simulink model "om2"  (Simulink 7.2)
(part 3 of 6)

      | Usage:                                                                                                                                                                                                                                    
      | Name the part with the desired filter module name.
      settings: AttributesFormatString=%<Tag>
  Y1_I : cdsFilt/Subsystem  Tag=cdsFilt  Description=|  SystemSampleTime=-1
      | Purpose:                                                                                                                                                                                                                                  
      | Standard CDS IIR filter module.                                                                                                                                                                                                           
      |                                                                                                                                                                                                                                           
      | Operation:                                                                                                                                                                                                                                
      | Consists of 10 second order section IIR filters, plus a ramped gain stage. In FE code, also provides pre-defined test points and excitation channel inputs. The filter coefficients are defined in the LIGO system using the 'foton' tool.
      |                                                                                                                                                                                                                                           
      | Usage:                                                                                                                                                                                                                                    
      | Name the part with the desired filter module name.
      settings: AttributesFormatString=%<Tag>
  Y1_MOUT : cdsEpicsOut/Subsystem  Tag=cdsEpicsOutput  Description=|  SystemSampleTime=-1
      | Purpose:                                          
      | Output a FE signal to an EPICS channel.           
      |                                                   
      | Operation:                                        
      | Takes input value and passes it to EPICS record.  
      |                                                   
      | Usage:                                            
      | Name the part with the desired EPICS rrecord name.
      settings: AttributesFormatString=%<Tag>
  Y1_OSC : cdsOsc/Subsystem  Tag=cdsOsc  Description=Oscillator  SystemSampleTime=-1
      settings: AttributesFormatString=%<Tag>
  Y1_OSC1 : cdsOsc/Subsystem  Tag=cdsOsc  Description=Oscillator  SystemSampleTime=-1
      settings: AttributesFormatString=%<Tag>
  Y1_PHASE : cdsPhaseDeg/Subsystem  Tag=cdsPhaseDeg  Description=Phase Rotator  SystemSampleTime=-1
      settings: AttributesFormatString=%<Tag>
  Y1_Q : cdsFilt/Subsystem  Tag=cdsFilt  Description=|  SystemSampleTime=-1
      | Purpose:                                                                                                                                                                                                                                  
      | Standard CDS IIR filter module.                                                                                                                                                                                                           
      |                                                                                                                                                                                                                                           
      | Operation:                                                                                                                                                                                                                                
      | Consists of 10 second order section IIR filters, plus a ramped gain stage. In FE code, also provides pre-defined test points and excitation channel inputs. The filter coefficients are defined in the LIGO system using the 'foton' tool.
      |                                                                                                                                                                                                                                           
      | Usage:                                                                                                                                                                                                                                    
      | Name the part with the desired filter module name.
      settings: AttributesFormatString=%<Tag>
  Y1_SIG : cdsFilt/Subsystem  Tag=cdsFilt  Description=|  SystemSampleTime=-1
      | Purpose:                                                                                                                                                                                                                                  
      | Standard CDS IIR filter module.                                                                                                                                                                                                           
      |                                                                                                                                                                                                                                           
      | Operation:                                                                                                                                                                                                                                
      | Consists of 10 second order section IIR filters, plus a ramped gain stage. In FE code, also provides pre-defined test points and excitation channel inputs. The filter coefficients are defined in the LIGO system using the 'foton' tool.
      |                                                                                                                                                                                                                                           
      | Usage:                                                                                                                                                                                                                                    
      | Name the part with the desired filter module name.
      settings: AttributesFormatString=%<Tag>
  Y1_X_COS : cdsFilt/Subsystem  Tag=cdsFilt  Description=|  SystemSampleTime=-1
      | Purpose:                                                                                                                                                                                                                                  
      | Standard CDS IIR filter module.                                                                                                                                                                                                           
      |                                                                                                                                                                                                                                           
      | Operation:                                                                                                                                                                                                                                
      | Consists of 10 second order section IIR filters, plus a ramped gain stage. In FE code, also provides pre-defined test points and excitation channel inputs. The filter coefficients are defined in the LIGO system using the 'foton' tool.
      |                                                                                                                                                                                                                                           
      | Usage:                                                                                                                                                                                                                                    
      | Name the part with the desired filter module name.
      settings: AttributesFormatString=%<Tag>
  Y1_X_SIN : cdsFilt/Subsystem  Tag=cdsFilt  Description=|  SystemSampleTime=-1
      | Purpose:                                                                                                                                                                                                                                  
      | Standard CDS IIR filter module.                                                                                                                                                                                                           
      |                                                                                                                                                                                                                                           
      | Operation:                                                                                                                                                                                                                                
      | Consists of 10 second order section IIR filters, plus a ramped gain stage. In FE code, also provides pre-defined test points and excitation channel inputs. The filter coefficients are defined in the LIGO system using the 'foton' tool.
      |                                                                                                                                                                                                                                           
      | Usage:                                                                                                                                                                                                                                    
      | Name the part with the desired filter module name.
      settings: AttributesFormatString=%<Tag>
  Y2_CLOCK : cdsFilt/Subsystem  Tag=cdsFilt  Description=|  SystemSampleTime=-1
      | Purpose:                                                                                                                                                                                                                                  
      | Standard CDS IIR filter module.                                                                                                                                                                                                           
      |                                                                                                                                                                                                                                           
      | Operation:                                                                                                                                                                                                                                
      | Consists of 10 second order section IIR filters, plus a ramped gain stage. In FE code, also provides pre-defined test points and excitation channel inputs. The filter coefficients are defined in the LIGO system using the 'foton' tool.
      |                                                                                                                                                                                                                                           
      | Usage:                                                                                                                                                                                                                                    
      | Name the part with the desired filter module name.
      settings: AttributesFormatString=%<Tag>
  Y2_I : cdsFilt/Subsystem  Tag=cdsFilt  Description=|  SystemSampleTime=-1
      | Purpose:                                                                                                                                                                                                                                  
      | Standard CDS IIR filter module.                                                                                                                                                                                                           
      |                                                                                                                                                                                                                                           
      | Operation:                                                                                                                                                                                                                                
      | Consists of 10 second order section IIR filters, plus a ramped gain stage. In FE code, also provides pre-defined test points and excitation channel inputs. The filter coefficients are defined in the LIGO system using the 'foton' tool.
      |                                                                                                                                                                                                                                           
      | Usage:                                                                                                                                                                                                                                    
      | Name the part with the desired filter module name.
      settings: AttributesFormatString=%<Tag>
  Y2_MOUT : cdsEpicsOut/Subsystem  Tag=cdsEpicsOutput  Description=|  SystemSampleTime=-1
      | Purpose:                                          
      | Output a FE signal to an EPICS channel.           
      |                                                   
      | Operation:                                        
      | Takes input value and passes it to EPICS record.  
      |                                                   
      | Usage:                                            
      | Name the part with the desired EPICS rrecord name.
      settings: AttributesFormatString=%<Tag>
  Y2_OSC : cdsOsc/Subsystem  Tag=cdsOsc  Description=Oscillator  SystemSampleTime=-1
      settings: AttributesFormatString=%<Tag>
  Y2_OSC1 : cdsOsc/Subsystem  Tag=cdsOsc  Description=Oscillator  SystemSampleTime=-1
      settings: AttributesFormatString=%<Tag>
  Y2_PHASE : cdsPhaseDeg/Subsystem  Tag=cdsPhaseDeg  Description=Phase Rotator  SystemSampleTime=-1
      settings: AttributesFormatString=%<Tag>
  Y2_Q : cdsFilt/Subsystem  Tag=cdsFilt  Description=|  SystemSampleTime=-1
      | Purpose:                                                                                                                                                                                                                                  
      | Standard CDS IIR filter module.                                                                                                                                                                                                           
      |                                                                                                                                                                                                                                           
      | Operation:                                                                                                                                                                                                                                
      | Consists of 10 second order section IIR filters, plus a ramped gain stage. In FE code, also provides pre-defined test points and excitation channel inputs. The filter coefficients are defined in the LIGO system using the 'foton' tool.
      |                                                                                                                                                                                                                                           
      | Usage:                                                                                                                                                                                                                                    
      | Name the part with the desired filter module name.
      settings: AttributesFormatString=%<Tag>
  Y2_SIG : cdsFilt/Subsystem  Tag=cdsFilt  Description=|  SystemSampleTime=-1
      | Purpose:                                                                                                                                                                                                                                  
      | Standard CDS IIR filter module.                                                                                                                                                                                                           
      |                                                                                                                                                                                                                                           
      | Operation:                                                                                                                                                                                                                                
      | Consists of 10 second order section IIR filters, plus a ramped gain stage. In FE code, also provides pre-defined test points and excitation channel inputs. The filter coefficients are defined in the LIGO system using the 'foton' tool.
      |                                                                                                                                                                                                                                           
      | Usage:                                                                                                                                                                                                                                    
      | Name the part with the desired filter module name.
      settings: AttributesFormatString=%<Tag>
  Y2_X_COS : cdsFilt/Subsystem  Tag=cdsFilt  Description=|  SystemSampleTime=-1
      | Purpose:                                                                                                                                                                                                                                  
      | Standard CDS IIR filter module.                                                                                                                                                                                                           
      |                                                                                                                                                                                                                                           
      | Operation:                                                                                                                                                                                                                                
      | Consists of 10 second order section IIR filters, plus a ramped gain stage. In FE code, also provides pre-defined test points and excitation channel inputs. The filter coefficients are defined in the LIGO system using the 'foton' tool.
      |                                                                                                                                                                                                                                           
      | Usage:                                                                                                                                                                                                                                    
      | Name the part with the desired filter module name.
      settings: AttributesFormatString=%<Tag>
  Y2_X_SIN : cdsFilt/Subsystem  Tag=cdsFilt  Description=|  SystemSampleTime=-1
      | Purpose:                                                                                                                                                                                                                                  
      | Standard CDS IIR filter module.                                                                                                                                                                                                           
      |                                                                                                                                                                                                                                           
      | Operation:                                                                                                                                                                                                                                
      | Consists of 10 second order section IIR filters, plus a ramped gain stage. In FE code, also provides pre-defined test points and excitation channel inputs. The filter coefficients are defined in the LIGO system using the 'foton' tool.
      |                                                                                                                                                                                                                                           
      | Usage:                                                                                                                                                                                                                                    
      | Name the part with the desired filter module name.
      settings: AttributesFormatString=%<Tag>
  T1P1 : Outport  OutDataType=sfix(16)  OutScaling=2^0
  T1Y1 : Outport  Port=2  OutDataType=sfix(16)  OutScaling=2^0
  T2P1 : Outport  Port=3  OutDataType=sfix(16)  OutScaling=2^0
  T2Y1 : Outport  Port=4  OutDataType=sfix(16)  OutScaling=2^0
  wires:
  P1_SIG/1 -> Product/1, Product1/1
  Product1/1 -> P1_X_COS/1
  Product/1 -> P1_X_SIN/1
  Y1_SIG/1 -> Product2/1, Product3/1
  Product3/1 -> Y1_X_COS/1
  Product2/1 -> Y1_X_SIN/1
  Ground1/1 -> Y1_OSC/1
  PD_IN/1 -> P1_MOUT/1, Y1_MOUT/1, P2_MOUT/1, Y2_MOUT/1
  P2_SIG/1 -> Product4/1, Product5/1
  Product5/1 -> P2_X_COS/1
  Product4/1 -> P2_X_SIN/1
  Ground2/1 -> P2_OSC/1
  Y2_SIG/1 -> Product6/1, Product7/1
  Product7/1 -> Y2_X_COS/1
  Product6/1 -> Y2_X_SIN/1
  Ground3/1 -> Y2_OSC/1
  P1_MOUT/1 -> P1_SIG/1
  Y1_MOUT/1 -> Y1_SIG/1
  P2_MOUT/1 -> P2_SIG/1
  Y2_MOUT/1 -> Y2_SIG/1
  P1_X_SIN/1 -> P1_PHASE/1
  P1_X_COS/1 -> P1_PHASE/2
  Y1_X_SIN/1 -> Y1_PHASE/1
  Y1_X_COS/1 -> Y1_PHASE/2
  P2_X_SIN/1 -> P2_PHASE/1
  P2_X_COS/1 -> P2_PHASE/2
  Y2_X_SIN/1 -> Y2_PHASE/1
  Y2_X_COS/1 -> Y2_PHASE/2
  P1_PHASE/1 -> P1_I/1
  P1_PHASE/2 -> P1_Q/1
  Y1_PHASE/1 -> Y1_I/1
  Y1_PHASE/2 -> Y1_Q/1
  P2_PHASE/1 -> P2_I/1
  P2_PHASE/2 -> P2_Q/1
  Y2_PHASE/1 -> Y2_I/1
  Y2_PHASE/2 -> Y2_Q/1
  P1_I/1 -> ACMTX/1
  P1_Q/1 -> ACMTX/2
  Y1_I/1 -> ACMTX/3
  Y1_Q/1 -> ACMTX/4
  Y2_Q/1 -> ACMTX/8
  Y2_I/1 -> ACMTX/7
  P2_Q/1 -> ACMTX/6
  P2_I/1 -> ACMTX/5
  Ground/1 -> P1_OSC/1
  P1_OSC/2 -> EXMTX/1, SINSW/2
  P1_OSC/3 -> EXMTX/2, COSSW/2
  Y1_OSC/2 -> EXMTX/3, SINSW/4
  Y1_OSC/3 -> EXMTX/4, COSSW/4
  P2_OSC/2 -> EXMTX/5, SINSW/6
  P2_OSC/3 -> EXMTX/6, COSSW/6
  EXMTX/1 -> P1_CLOCK/1
  EXMTX/2 -> Y1_CLOCK/1
  EXMTX/3 -> P2_CLOCK/1
  EXMTX/4 -> Y2_CLOCK/1
  Y2_OSC/2 -> EXMTX/7, SINSW/8
  Y2_OSC/3 -> EXMTX/8, COSSW/8
  Y2_OSC/1 -> Terminator3/1
  P2_OSC/1 -> Terminator2/1
  Y1_OSC/1 -> Terminator1/1
  P1_OSC/1 -> Terminator/1
  QPD3P/1 -> QPDASC/1, Mux/1
  QPD3Y/1 -> QPDASC/2, Mux/2
  QPD4P/1 -> Mux/3, QPDASC/3
  QPD4Y/1 -> QPDASC/4, Mux/4
  QPDASC/1 -> QPOS_Y/1, QPOS_Y_B/1
  QPDASC/3 -> QANG_Y/1, QANG_Y_B/1
  QPDASC/4 -> QANG_X/1, QANG_X_B/1
  ACMTX/1 -> DPOS_Y/1, DPOS_Y_B/1
  ACMTX/2 -> DPOS_X/1, DPOS_X_B/1
  ACMTX/3 -> DANG_Y/1, DANG_Y_B/1
  Sum4/1 -> BLENDGAIN/1
  Sum5/1 -> BLENDGAIN/2
  Sum6/1 -> BLENDGAIN/3
  Sum7/1 -> BLENDGAIN/4
  DPOS_Y/1 -> DITHERGAIN/1
  DPOS_X/1 -> DITHERGAIN/2
  DANG_Y/1 -> DITHERGAIN/3
  DANG_X/1 -> DITHERGAIN/4
  QPOS_Y/1 -> QPDGAIN/1
  QPOS_X/1 -> QPDGAIN/2
  QANG_Y/1 -> QPDGAIN/3
  QANG_X/1 -> QPDGAIN/4
  Mux/1 -> WAISTBASIS/1
  WAISTBASIS/1 -> Demux/1
  WAIST_X/1 -> Terminator4/1
  WAIST_Y/1 -> Terminator5/1
  WAIST_PIT/1 -> Terminator6/1
  WAIST_YAW/1 -> Terminator7/1
  Demux/1 -> WAIST_X/1
  Demux/2 -> WAIST_Y/1
  Demux/3 -> WAIST_PIT/1
  Demux/4 -> WAIST_YAW/1
  QPDASC/2 -> QPOS_X/1, QPOS_X_B/1
  MASTERGAIN/1 -> POS_Y/1
  MASTERGAIN/2 -> POS_X/1
  MASTERGAIN/3 -> ANG_Y/1
  MASTERGAIN/4 -> ANG_X/1
  Sum10/1 -> MASTERGAIN/3
  Sum11/1 -> MASTERGAIN/4
  QPD1_P_SIG/1 -> Product8/1, Product9/1
  Product9/1 -> QPD1_P_C/1
  Product8/1 -> QPD1_P_S/1
  QPD1_P_MOUT/1 -> QPD1_P_SIG/1
  QPD1_P_S/1 -> QPD1_P_PHASE/1
  QPD1_P_C/1 -> QPD1_P_PHASE/2
  QPD1_P_PHASE/1 -> QPD1_P_I/1
  QPD1_P_PHASE/2 -> QPD1_P_Q/1
  QPD1_Y_SIG/1 -> Product10/1, Product11/1
  Product11/1 -> QPD1_Y_C/1
  Product10/1 -> QPD1_Y_S/1
  QPD1_Y_MOUT/1 -> QPD1_Y_SIG/1
  QPD1_Y_S/1 -> QPD1_Y_PHASE/1
  QPD1_Y_C/1 -> QPD1_Y_PHASE/2
  QPD1_Y_PHASE/1 -> QPD1_Y_I/1
  QPD1_Y_PHASE/2 -> QPD1_Y_Q/1
  QPD1Y/1 -> QPD1_Y_MOUT/1
  QPD1P/1 -> QPD1_P_MOUT/1
  LSC_SIN/1 -> Product8/2, Product10/2, Product14/2, Product12/2
  LSC_COS/1 -> Product9/2, Product11/2, Product15/2, Product13/2
  QPD1_Y_Q/1 -> Terminator9/1
  QPD1_P_Q/1 -> Terminator8/1
  QPD1_Y_I/1 -> RDASC/2
  QPD1_P_I/1 -> RDASC/1
  QPD2_Y_SIG/1 -> Product12/1, Product13/1
  Product13/1 -> QPD2_Y_C/1
  Product12/1 -> QPD2_Y_S/1
  QPD2_Y_MOUT/1 -> QPD2_Y_SIG/1
  QPD2_Y_S/1 -> QPD2_Y_PHASE/1
  QPD2_Y_C/1 -> QPD2_Y_PHASE/2
  QPD2_Y_PHASE/1 -> QPD2_Y_I/1
  QPD2_Y_PHASE/2 -> QPD2_Y_Q/1
  QPD2_Y_Q/1 -> Terminator13/1
  QPD2_Y_I/1 -> RDASC/4
  QPD2_P_SIG/1 -> Product14/1, Product15/1
  Product15/1 -> QPD2_P_C/1
  Product14/1 -> QPD2_P_S/1
  QPD2_P_MOUT/1 -> QPD2_P_SIG/1
  QPD2_P_S/1 -> QPD2_P_PHASE/1
  QPD2_P_C/1 -> QPD2_P_PHASE/2
  QPD2_P_PHASE/1 -> QPD2_P_I/1
  QPD2_P_PHASE/2 -> QPD2_P_Q/1
  QPD2_P_Q/1 -> Terminator15/1
  QPD2_P_I/1 -> RDASC/3
  QPD2Y/1 -> QPD2_Y_MOUT/1
  QPD2P/1 -> QPD2_P_MOUT/1
  RDASC/1 -> RPOS_Y/1, RPOS_Y_B/1
  RDASC/2 -> RPOS_X/1, RPOS_X_B/1
  RDASC/3 -> RANG_Y/1, RANG_Y_B/1
  RDASC/4 -> RANG_X/1, RANG_X_B/1
  RPOS_Y/1 -> RDAGAIN/1
  RPOS_X/1 -> RDAGAIN/2
  RANG_Y/1 -> RDAGAIN/3
  RANG_X/1 -> RDAGAIN/4
  Sum9/1 -> MASTERGAIN/2
  Sum8/1 -> MASTERGAIN/1
  RDAGAIN/1 -> Sum8/1
  RDAGAIN/2 -> Sum9/1
  RDAGAIN/3 -> Sum10/1
  RDAGAIN/4 -> Sum11/1
  BLENDGAIN/1 -> Sum8/2
  BLENDGAIN/2 -> Sum9/2
  BLENDGAIN/3 -> Sum10/2
  BLENDGAIN/4 -> Sum11/2
  QPDGAIN/1 -> Sum8/3
  QPDGAIN/2 -> Sum9/3
  QPDGAIN/3 -> Sum10/3
  QPDGAIN/4 -> Sum11/3
  DITHERGAIN/1 -> Sum8/4
  DITHERGAIN/2 -> Sum9/4
  DITHERGAIN/4 -> Sum11/4
  DITHERGAIN/3 -> Sum10/4
  ACMTX/4 -> DANG_X/1, DANG_X_B/1
  P1_CLOCK/1 -> Sum1/2
  POS_Y/1 -> Sum1/1
  Sum1/1 -> T1P1/1
  Y1_CLOCK/1 -> Sum2/2
  Sum2/1 -> T1Y1/1
  POS_X/1 -> Sum2/1
  Sum3/1 -> T2P1/1
  Sum12/1 -> T2Y1/1
  ANG_Y/1 -> Sum3/1
  ANG_X/1 -> Sum12/1
  P2_CLOCK/1 -> Sum3/2
  Y2_CLOCK/1 -> Sum12/2
  RPOS_Y_B/1 -> Sum4/1
  QPOS_Y_B/1 -> Sum4/2
  DPOS_Y_B/1 -> Sum4/3
  RPOS_X_B/1 -> Sum5/1
  QPOS_X_B/1 -> Sum5/2
  DPOS_X_B/1 -> Sum5/3
  RANG_Y_B/1 -> Sum6/1
  QANG_Y_B/1 -> Sum6/2
  DANG_Y_B/1 -> Sum6/3
  DANG_X_B/1 -> Sum7/3
  QANG_X_B/1 -> Sum7/2
  RANG_X_B/1 -> Sum7/1
  Ground5/1 -> Y1_OSC1/1
  Ground6/1 -> P2_OSC1/1
  Ground7/1 -> Y2_OSC1/1
  Ground4/1 -> P1_OSC1/1
  Y2_OSC1/1 -> Terminator14/1
  P2_OSC1/1 -> Terminator12/1
  Y1_OSC1/1 -> Terminator11/1
  P1_OSC1/1 -> Terminator10/1
  P1_OSC1/2 -> SINSW/1
  Y1_OSC1/2 -> SINSW/3
  P2_OSC1/2 -> SINSW/5
  Y2_OSC1/2 -> SINSW/7
  SINSW/1 -> Product/2
  P1_OSC1/3 -> COSSW/1
  Y1_OSC1/3 -> COSSW/3
  P2_OSC1/3 -> COSSW/5
  Y2_OSC1/3 -> COSSW/7
  COSSW/1 -> Product1/2
  SINSW/2 -> Product2/2
  SINSW/3 -> Product4/2
  SINSW/4 -> Product6/2
  COSSW/2 -> Product3/2
  COSSW/3 -> Product5/2
  COSSW/4 -> Product7/2
  SINSW/5 -> SINSW_MON/1
  COSSW/5 -> COSSW_MON/1
  COSSW_MON/1 -> Terminator16/1
  SINSW_MON/1 -> Terminator17/1
